simulink model "Weighted_PID"  (R2015a)
settings: Solver=ode3  StartTime=0.0  StopTime=inf  FixedStep=1e-3  RelTol=1e-3
values from neighbouring files (symbols this model uses):
  conversion_V2mm = 17.8/(3540-260)    (= 0.00542682926829)    [Datasheet.m]    (also in setup.m)
  deltaVals = [1 1.48717948718 1.97435897436 2.46153846154 2.94871794872 3.4358974359 3.92307692308 4.41025641026 4.89743589744 5.38461538462 5.87179487179 6.35897435897 ... (40 elements, 1x40)]    [Execution_params.mat]    (also in Vals_Gen.m = linspace (1, 20, length(deltas)))
  Kvals = [31.6321598713 27.3610646357 24.1061588491 21.5433370653 19.4730767023 17.7658256591 16.3338022856 15.1154164856 14.0661792785 13.1531526871 12.3514294003 11.6418259188 ... (40 elements, 1x40)]    [Execution_params.mat]    (also in Vals_Gen.m = zeros(1, n))
libraries: PoliArd x6, dsparch4 x3, simulink x2
settings Model: ExtModeTrigDuration=2  Creator=User  LastModifiedBy=User
settings OptimizationCC: OptimizeModelRefInitCode=on  LifeSpan=1
settings DebuggingCC: UnderspecifiedInitializationDetection=Classic  MergeDetectMultiDrivingBlocksExec=none
settings HardwareCC: ProdLargestAtomicInteger=Long  ProdLargestAtomicFloat=Double  ProdEndianess=LittleEndian  ProdHWDeviceType=ARM Compatible->ARM Cortex
settings RTWCC: SystemTargetFile=realtime.tlc  GenerateMakefile=off  TemplateMakefile=realtime.tmf  Description=Run on Target Hardware  RTWVerbose=off
settings ERTTargetCC: CombineOutputUpdateFcns=off  ExtModeTransport=3  ExtModeMexFile=ext_serial_win32_comm_rtt  ExtModeMexArgs=0 1 9600  ERTSrcFileBannerTemplate=realtime_code_template.cgt  ERTHdrFileBannerTemplate=realtime_code_template.cgt  ERTDataSrcFileTemplate=realtime_code_template.cgt  ERTDataHdrFileTemplate=realtime_code_template.cgt  ERTCustomFileTemplate=realtime_file_process.tlc

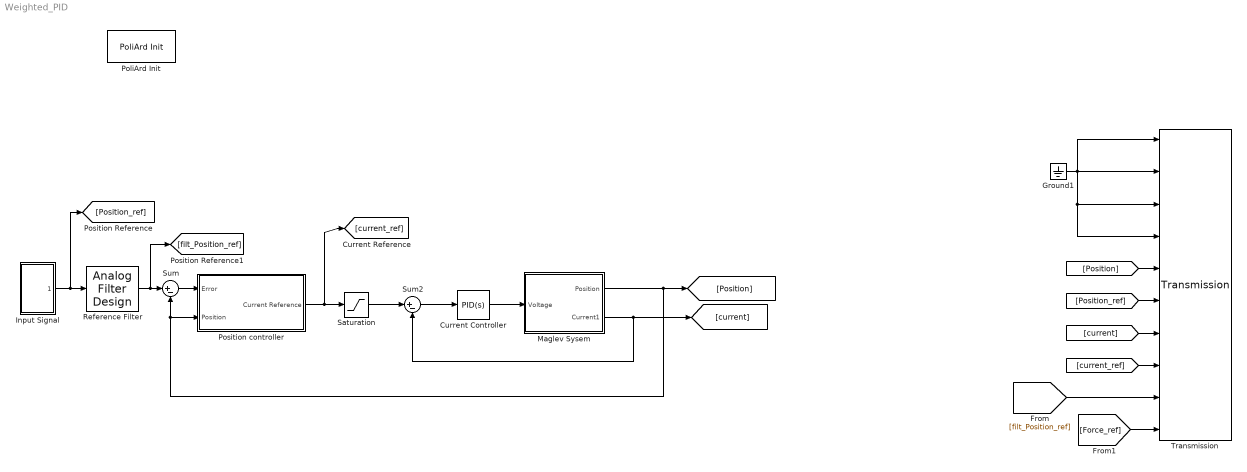
== system Weighted_PID ==
  Current Controller : simulink/Continuous/PID Controller  Controller=PID  TimeDomain=Continuous-time  SampleTime=-1  IntegratorMethod=Forward Euler  FilterMethod=Forward Euler  Form=Parallel  UseFilter=on  ControllerParametersSource=internal  P=35  I=350  D=0  N=0  InitialConditionSource=internal  InitialConditionForIntegrator=0  InitialConditionForFilter=0  ExternalReset=none  LimitOutput=on  UpperSaturationLimit=24  LowerSaturationLimit=-24  LinearizeAsGain=on  AntiWindupMode=none  Kb=1  TrackingMode=off  Kt=1  PParamMin=[]  PParamMax=[]  IParamMin=[]  IParamMax=[]  DParamMin=[]  DParamMax=[]  NParamMin=[]  NParamMax=[]  KbParamMin=[]  KbParamMax=[]  KtParamMin=[]  KtParamMax=[]  POutMin=[]  POutMax=[]  IOutMin=[]  IOutMax=[]  DOutMin=[]  DOutMax=[]  NOutMin=[]  NOutMax=[]  KbOutMin=[]  KbOutMax=[]  KtOutMin=[]  KtOutMax=[]  IntegratorOutMin=[]  IntegratorOutMax=[]  FilterOutMin=[]  FilterOutMax=[]  SumOutMin=[]  SumOutMax=[]  SumI1OutMin=[]  SumI1OutMax=[]  SumI2OutMin=[]  SumI2OutMax=[]  SumI3OutMin=[]  SumI3OutMax=[]  SumDOutMin=[]  SumDOutMax=[]  SaturationOutMin=[]  SaturationOutMax=[]  IntegratorContinuousStateAttributes=''  IntegratorStateMustResolveToSignalObject=off  IntegratorRTWStateStorageClass=Auto  FilterContinuousStateAttributes=''  FilterStateMustResolveToSignalObject=off  FilterRTWStateStorageClass=Auto  DifferentiatorICPrevScaledInput=0  DifferentiatorOutMin=[]  DifferentiatorOutMax=[]
  Ground1 : Ground
  Input Signal : Subsystem
  Maglev Sysem : Subsystem
  PoliArd Init : PoliArd/PoliArd Init
  Position controller : Subsystem
  Reference Filter : dsparch4/Analog Filter Design  method=Butterworth  filttype=Lowpass  N=1  Wlo=10  Whi=80  Rp=2  Rs=40
  Saturation : Saturate  UpperLimit=10  LowerLimit=0
  Sum : Sum  Inputs=|+-
  Sum2 : Sum  Inputs=|+-
  Transmission : PoliArd/Transmission  sample_freq=100  sig_to_send=6
  wires:
  Sum2/1 -> Current Controller/1
  Ground1/1 -> Transmission/4, Transmission/3, Transmission/1, Transmission/2
  [Position_ref] -> Transmission/6
  Sum/1 -> Position controller/1(Error)
  Maglev Sysem/1(Position) -> Sum/2, Position controller/2(Position), [Position]
  Position controller/1(Current Reference) -> Saturation/1, [current_ref]
  Current Controller/1 -> Maglev Sysem/1(Voltage)
  Maglev Sysem/2(Current1) -> Sum2/2, [current]
  [Position] -> Transmission/5
  [current] -> Transmission/7
  [current_ref] -> Transmission/8
  Saturation/1 -> Sum2/1
  [filt_Position_ref] -> Transmission/9
  Input Signal/1(Signal) -> Reference Filter/1, [Position_ref]
  [Force_ref] -> Transmission/10
  Reference Filter/1 -> [filt_Position_ref], Sum/1

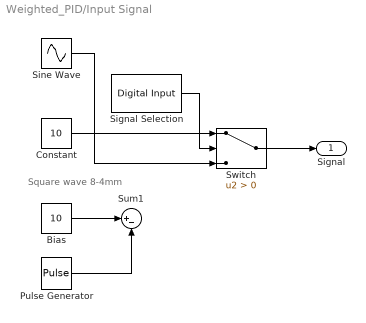
== system Weighted_PID/Input Signal ==
  note: Square wave 8-4mm
  Bias : Constant  Value=10
  Constant : Constant  Value=10
  Pulse Generator : DiscretePulseGenerator  PulseType=Time based  Amplitude=4  Period=4  PulseWidth=50
  Signal Selection : PoliArd/Digital Input  DI_pin=2  DIsample=-1
  Sine Wave : Sin  Amplitude=2  Bias=8  Frequency=3  SampleTime=0
  Sum1 : Sum  Inputs=|+-
  Switch : Switch  Criteria=u2 > Threshold
  Signal : Outport
  wires:
  Pulse Generator/1 -> Sum1/2
  Bias/1 -> Sum1/1
  Constant/1 -> Switch/1
  Switch/1 -> Signal/1
  Signal Selection/1 -> Switch/2
  Sine Wave/1 -> Switch/3

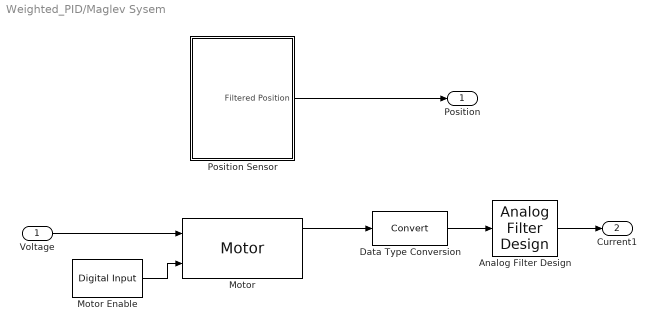
== system Weighted_PID/Maglev Sysem ==
  Voltage : Inport
  Analog Filter Design : dsparch4/Analog Filter Design  method=Butterworth  filttype=Lowpass  N=1  Wlo=150  Whi=80  Rp=2  Rs=40
  Data Type Conversion : DataTypeConversion
  Motor : PoliArd/Motor  MotorID=2  DC_bus_mask=24  dt_mot=-1
  Motor Enable : PoliArd/Digital Input  DI_pin=3  DIsample=-1
  Position Sensor : Subsystem
  Position : Outport
  Current1 : Outport  Port=2
  wires:
  Motor Enable/1 -> Motor/2
  Voltage/1 -> Motor/1
  Position Sensor/1(Filtered Position) -> Position/1
  Data Type Conversion/1 -> Analog Filter Design/1
  Motor/1 -> Data Type Conversion/1
  Analog Filter Design/1 -> Current1/1

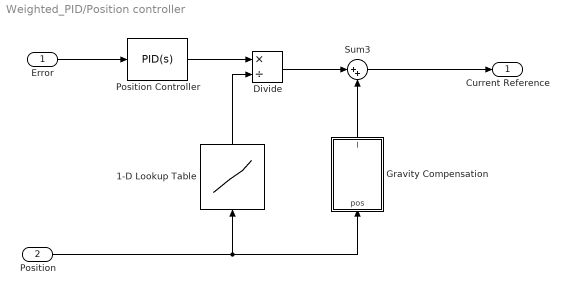
== system Weighted_PID/Position controller ==
  Error : Inport
  Position : Inport  Port=2
  1-D Lookup Table : Lookup_n-D  NumberOfTableDimensions=1  BreakpointsForDimension1=deltaVals  Table=Kvals  InternalRulePriority=Speed  RndMeth=Simplest  InputSameDT=on
  Divide : Product  Inputs=*/
  Gravity Compensation : MATLAB Function  TreatAsAtomicUnit=on
  Position Controller : simulink/Continuous/PID Controller  Controller=PID  TimeDomain=Continuous-time  SampleTime=-1  IntegratorMethod=Forward Euler  FilterMethod=Forward Euler  Form=Parallel  UseFilter=on  ControllerParametersSource=internal  P=-2  I=-40  D=-0.15  N=100  InitialConditionSource=internal  InitialConditionForIntegrator=0  InitialConditionForFilter=0  ExternalReset=none  LimitOutput=on  UpperSaturationLimit=8  LowerSaturationLimit=-8  LinearizeAsGain=on  AntiWindupMode=back-calculation  Kb=1  TrackingMode=off  Kt=1  PParamMin=[]  PParamMax=[]  IParamMin=[]  IParamMax=[]  DParamMin=[]  DParamMax=[]  NParamMin=[]  NParamMax=[]  KbParamMin=[]  KbParamMax=[]  KtParamMin=[]  KtParamMax=[]  POutMin=[]  POutMax=[]  IOutMin=[]  IOutMax=[]  DOutMin=[]  DOutMax=[]  NOutMin=[]  NOutMax=[]  KbOutMin=[]  KbOutMax=[]  KtOutMin=[]  KtOutMax=[]  IntegratorOutMin=[]  IntegratorOutMax=[]  FilterOutMin=[]  FilterOutMax=[]  SumOutMin=[]  SumOutMax=[]  SumI1OutMin=[]  SumI1OutMax=[]  SumI2OutMin=[]  SumI2OutMax=[]  SumI3OutMin=[]  SumI3OutMax=[]  SumDOutMin=[]  SumDOutMax=[]  SaturationOutMin=[]  SaturationOutMax=[]  IntegratorContinuousStateAttributes=''  IntegratorStateMustResolveToSignalObject=off  IntegratorRTWStateStorageClass=Auto  FilterContinuousStateAttributes=''  FilterStateMustResolveToSignalObject=off  FilterRTWStateStorageClass=Auto  DifferentiatorICPrevScaledInput=0  DifferentiatorOutMin=[]  DifferentiatorOutMax=[]
  Sum3 : Sum  Inputs=|++
  Current Reference : Outport
  wires:
  Position Controller/1 -> Divide/1
  1-D Lookup Table/1 -> Divide/2
  Error/1 -> Position Controller/1
  Gravity Compensation/1(I) -> Sum3/2
  Position/1 -> 1-D Lookup Table/1, Gravity Compensation/1(pos)
  Divide/1 -> Sum3/1
  Sum3/1 -> Current Reference/1

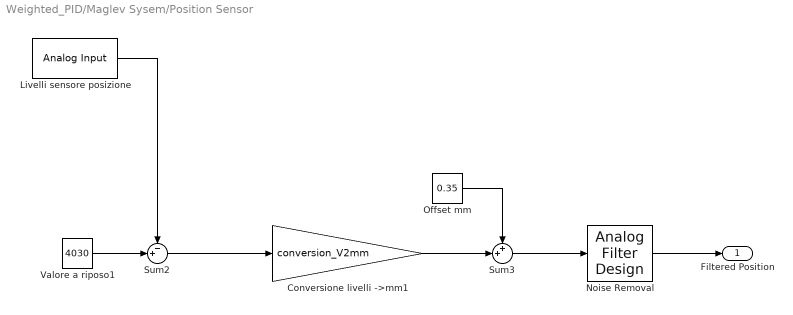
== system Weighted_PID/Maglev Sysem/Position Sensor ==
  Conversione livelli ->mm1 : Gain  Gain=conversion_V2mm
  "Livelli sensore posizione " : PoliArd/Analog Input  AIpin_mask=2  AIsample=-1
  Noise Removal : dsparch4/Analog Filter Design  method=Butterworth  filttype=Lowpass  N=1  Wlo=85  Whi=80  Rp=2  Rs=40
  Offset mm : Constant  Value=0.35
  Sum2 : Sum  Inputs=-+|
  Sum3 : Sum  Inputs=++|
  Valore a riposo1 : Constant  Value=4030
  Filtered Position : Outport
  wires:
  "Livelli sensore posizione "/1 -> Sum2/1
  Valore a riposo1/1 -> Sum2/2
  Sum2/1 -> Conversione livelli ->mm1/1
  Conversione livelli ->mm1/1 -> Sum3/2
  Sum3/1 -> Noise Removal/1
  Offset mm/1 -> Sum3/1
  Noise Removal/1 -> Filtered Position/1

== matlab function Weighted_PID/Position controller/Gravity Compensation ==
  data: I output; pos input
function I = fcn(pos)
q=0.1139;
m = 0.1932;
I=pos*m+q;

end
